simulink model "x2a2"  (R2024b)
settings: Solver=ode2  StartTime=0.0  StopTime=25  FixedStep=0.01  RelTol=1e-3
settings Model: Creator=john  LastModifiedBy=john

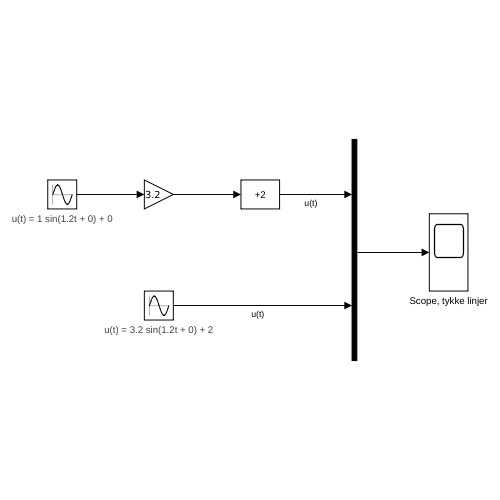
[thumbnail: Simulink's stored preview of the top-level diagram]
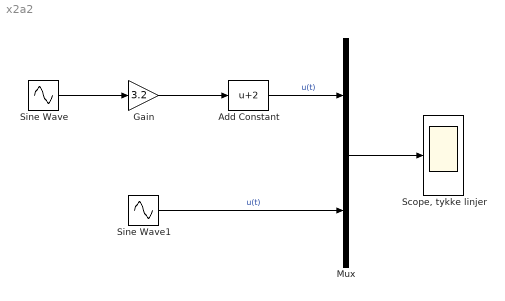
== system x2a2 ==
  Add Constant : Bias  Bias=2  SaturateOnIntegerOverflow=off
  Gain : Gain  Gain=3.2
  Mux : Mux  Inputs=2
  "Scope, tykke linjer" : Scope
  Sine Wave : Sin  Frequency=1.2  SampleTime=0
      settings: AttributesFormatString=u(t) = %<Amplitude> sin(%<Frequency>t + %<Phase>) + %<Bias>
  Sine Wave1 : Sin  Amplitude=3.2  Bias=2  Frequency=1.2  SampleTime=0
      settings: AttributesFormatString=u(t) = %<Amplitude> sin(%<Frequency>t + %<Phase>) + %<Bias>
  wires:
  Sine Wave/1 -> Gain/1
  Gain/1 -> Add Constant/1
  Add Constant/1 -> Mux/1  "u(t)"
  Sine Wave1/1 -> Mux/2  "u(t)"
  Mux/1 -> "Scope, tykke linjer"/1
